simulink model "distributive4"  (R2022b)
settings: Solver=ode8  StartTime=0.0  StopTime=0.25  FixedStep=0.0001  RelTol=1e-3
values from neighbouring files (symbols this model uses):
  A = [a11,0;0,a22]    [distributive3.m]    (also in neurobserver4.m = [1 1;1 2])
  alpha = 0.9e-6    (= 9e-07)    [distributive3.m]
  amp = 80e-6    (= 8e-05)    [distributive3.m]
  angvel = (2*pi)*30    (= 188.495559215)    [distributive3.m]
  B = [b11,0;0,b22]    [distributive3.m]    (also in neurobserver4.m = 1000)
  beta = 0.008    [distributive3.m]
  C = [1,0]    [distributive3.m]
  C_bar = [1,0]    [distributive3.m]    (also in neurobserver4.m = [1,0;0,1])
  d_p = 1.6e-6    (= 1.6e-06)    [distributive3.m]
  fase = 2*pi/10    (= 0.628318530718)    [distributive3.m]
  G = S\C_bar'    [distributive3.m]    (also in neurobserver4.m)
  gamma = 0.008    [distributive3.m]
  Gamma = [0,-B;0 0]    [distributive3.m]    (also in neurobserver4.m = [ 0 , -B ; 0 , 0 ])
  h = legend('Closed-loop response map $(y_d,y)$')    [distributive3.m]    (also in neurobserver4.m = legend('$(y_r,y)$ for $x=7.5$, $f=1Hz$','$(y_r,y)$ for $x=15)
  h_i = 2e-6    (= 2e-06)    [distributive3.m]
  k1 = 7    [distributive3.m]    (also in neurobserver4.m)
  k2 = 7    [distributive3.m]    (also in neurobserver4.m)
  kappa1 = 4e3    (= 4000)    [distributive3.m]    (also in neurobserver4.m = 120)
  L = 20000    [distributive3.m]
  S = [s11,s12;s21,s22]    [distributive3.m]    (also in neurobserver4.m = [1/theta,B/theta^2;B/theta^2,(2*B^2)/theta^3])
  V = learning.V    [neurobserver4.m]
  W = learning.W    [neurobserver4.m]
  x1 = e(2)    [distributive3.m]
  x2 = e(5)    [distributive3.m]
  y_i = -3e-6    (= -3e-06)    [distributive3.m]
undefined symbols (not defined in the file or in its folder): freq, Gamma_c, Y
(part 3 of 3)

== matlab function distributive4/observer10 ==
  data: z_hat input; y input; h_d input; C_bar parameter; S parameter; Gamma parameter; hZ input; z_hat_dot output; V parameter; W parameter
function z_hat_dot   = fcn(z_hat,y,h_d,C_bar,S,Gamma,hZ,V,W)
Y_hat=C_bar'*z_hat;
z=[y;h_d];
Y=C_bar'*z;

sigma = sig_fn(V*hZ);                                              % (8x1) = (8x8)*(8x1)
g_hat = W*sigma;                                                       % hg = (2x1) = (2x8)*(8x1)
G= S\C_bar;
z_hat_dot=Gamma*z_hat + g_hat + G*(Y-Y_hat); %G*C_bar*(z-z_hat); %
end

function [sigvec] = sig_fn(x_vec)
    sigvec = zeros(length(x_vec), 1);
    for i = 1:length(x_vec)
        sigvec(i, 1) = 2/(1 + exp(-2*x_vec(i, 1))) - 1;
    end
end

== matlab function distributive4/observer9 ==
  data: z_hat input; y input; h_d input; C_bar parameter; S parameter; Gamma parameter; hZ input; z_hat_dot output; V parameter; W parameter
function z_hat_dot   = fcn(z_hat,y,h_d,C_bar,S,Gamma,hZ,V,W)
z=[y;h_d];
z_tilde=z-z_hat;

sigma = sig_fn(V*hZ);                                              % (8x1) = (8x8)*(8x1)
g_hat = W*sigma;                                                       % hg = (2x1) = (2x8)*(8x1)
G= S\C_bar;
z_hat_dot=Gamma*z_hat + g_hat + G*(C_bar'*z_tilde); %G*C_bar*(z-z_hat); %
end

function [sigvec] = sig_fn(x_vec)
    sigvec = zeros(length(x_vec), 1);
    for i = 1:length(x_vec)
        sigvec(i, 1) = 2/(1 + exp(-2*x_vec(i, 1))) - 1;
    end
end

== matlab function distributive4/u_ref_dot10 ==
  data: h_d_ref input; z_hat input; u_ref_dot output size=1; alpha parameter size=1; k1 parameter size=1; k2 parameter size=1; x input; L parameter
function u_ref_dot = fcn(h_d_ref,z_hat,alpha,k1,k2,x,L)
h_d_hat=z_hat(2);
% syms c1 c2 k1 k2 alfa betta rho sigma

e = h_d_hat - h_d_ref;
alpha_d=alpha*(x/L)^2;

u_ref_dot=(1/alpha_d)*(k1*sign(e)*sqrt(abs(e)) + k2*e);
%u_ref_dot= k1*sign(e) + k2*e; %este es el ùnico que sí controla el modelo de micky con A_h=0.9e-6

== matlab function distributive4/u_ref_dot11 ==
  data: h_d_ref input; z_hat input; u_ref_dot output size=1; alpha parameter size=1; k1 parameter size=1; k2 parameter size=1; x input; L parameter
function u_ref_dot = fcn(h_d_ref,z_hat,alpha,k1,k2,x,L)
h_d_hat=z_hat(2);
% syms c1 c2 k1 k2 alfa betta rho sigma

e = h_d_hat - h_d_ref;
alpha_d=alpha*(x/L)^2;

u_ref_dot=(1/alpha_d)*(k1*sign(e)*sqrt(abs(e)) + k2*e);
%u_ref_dot= k1*sign(e) + k2*e; %este es el ùnico que sí controla el modelo de micky con A_h=0.9e-6

== matlab function distributive4/v10 ==
  data: d_d input; v output; u input; h_d input
function v = fcn(d_d,u,h_d)

v=d_d*u-h_d;

== matlab function distributive4/Subsystem10/y3 ==
  data: y output; v input; Y input; Y_dot output; A parameter; B parameter; C parameter; t input
function [y,Y_dot] = fcn(v,Y, A, B, C,t)

delta_y = [(30)*t;0];
Y_dot = A*Y + B*v + delta_y;
y=C*Y;

== matlab function distributive4/v11 ==
  data: d_d input; v output; u input; h_d input
function v = fcn(d_d,u,h_d)

v=d_d*u-h_d;

== matlab function distributive4/y12 ==
  data: y output; v input; Y input; Y_dot output; A parameter; B parameter; C parameter
function [y,Y_dot] = fcn(v,Y, A, B, C)
Y_dot=A*Y+B*v;
y=C*Y;

== matlab function distributive4/y13 ==
  data: y output; v input; Y input; Y_dot output; A parameter; B parameter; C parameter
function [y,Y_dot] = fcn(v,Y, A, B, C)
Y_dot=A*Y+B*v;
y=C*Y;

== matlab function distributive4/disturbances ==
  data: t input; delta output
function delta = dist(t)

delta_x = 30e-6; %0;
%delta_h = (25e-6)*sin(t); %0; %2*sin(t);

delta = delta_x;

== matlab function distributive4/dist_vars25/disturbances ==
  data: t input; delta output
function delta = dist(t)


delta_h = (25e-6)*sin(t); %2*sin(t);

delta = delta_h;

== matlab function distributive4/disturbances1 ==
  data: t input; delta output
function delta = dist(t)

delta_x = 30e-6; %0;
%delta_h = (25e-6)*sin(t); %0; %2*sin(t);

delta = delta_x;

== matlab function distributive4/dist_vars24/disturbances ==
  data: t input; delta output
function delta = dist(t)


delta_h = (25e-6)*sin(t); %2*sin(t);

delta = delta_h;

== matlab function distributive4/Subsystem2/Subsystem4/estimator ==
  data: h input; y_d_hat output; h_dot output; h_d_hat output; L parameter; u input; u_dot input; d_p parameter; d_d_hat output; alpha parameter; gamma parameter; x input; beta parameter
function [y_d_hat,h_dot,h_d_hat,d_d_hat]  = fcn(h,L, u,u_dot,d_p, alpha, gamma,x, beta)

d_d_hat = d_p*(x/L)^2;
h_dot = alpha*u_dot - beta*abs(u_dot)*h - gamma*u_dot*abs(h);
%h_d_dot = h_dot*(x/L)^2;
%h_d_hat = h*(x/L)^2;
%u_hat = (y_L + h_d_hat)/d_d_hat;
h_d_hat = h*(x/L)^2;
y_d_hat = d_d_hat*u -h_d_hat;




%h_d=h*(x/L)^2;
%

== matlab function distributive4/Subsystem2/Subsystem4/measurements/MATLAB Function1 ==
  data: h input; u input; y_L output; d_p parameter
function y_L = fcn(h,u,d_p)


y_L = d_p*u-h;

== matlab function distributive4/Subsystem2/Subsystem4/measurements/MATLAB Function5 ==
  data: u_dot input; h_dot output; h input; alpha parameter; gamma parameter; beta parameter
function h_dot = fcn(u_dot,h,alpha, gamma, beta)

h_dot = alpha*u_dot - beta*abs(u_dot)*h - gamma*u_dot*abs(h);

== matlab function distributive4/Subsystem/dist_vars32/MATLAB Function ==
  data: x input; L parameter; d_p parameter; d_d output
function d_d   = fcn(x,L, d_p)

d_d = (x/L)*(x/L)*d_p;

== matlab function distributive4/Subsystem/dist_vars32/MATLAB Function5 ==
  data: u_dot input; h_dot output; h input; x input; alpha parameter; gamma parameter; beta parameter; L parameter; h_d output; t input
function [h_dot,h_d] = fcn(u_dot,h,x,alpha, gamma, beta,L,t)

delta_h=25*t;
h_dot = alpha*u_dot - beta*abs(u_dot)*h - gamma*u_dot*abs(h) + delta_h; % ****
h_d=h*(x/L)^2;     % ****
%h_d_dot = h_dot*(x/L)^2;

% function [h_dot,h_d_dot]  = fcn(u_dot,h,x,alpha, gamma, beta,L,t)

% delta_h=25*t;
% h_dot = alpha*u_dot - beta*abs(u_dot)*h - gamma*u_dot*abs(h) + delta_h;
% h_d_dot = h_dot*(x/L)^2;
%h_d=h*(x/L)^2;

== matlab function distributive4/Subsystem2/inv D3 ==
  data: y_ref input; Y_dot input; A parameter; B parameter; v_ref output; Y output; C parameter
%function h_d_ref = fcn(y,y_ref_dot,d_d,u, A, B)

%y_tilde=y_hat-y_ref;
%h_d_ref=(1/B)*(A*y -y_ref_dot +B*d_d*u);

function [v_ref,Y]  = fcn(y_ref,Y_dot, A, B, C)

Y=y_ref/C;
v_ref = (Y_dot-A*Y)/B;

== matlab function distributive4/dist_vars3/MATLAB Function ==
  data: x input; L parameter; d_p parameter; d_d output
function d_d   = fcn(x,L, d_p)

d_d = (x/L)*(x/L)*d_p;

== matlab function distributive4/Subsystem2/inv v3 ==
  data: v input; h_d input; u_ref output size=1; d_d input size=1
%function u_ref_dot = fcn(h_d_hat,h_d_ref,alpha,k1,k2)
function u_ref = fcn(v,h_d,d_d)
% syms c1 c2 k1 k2 alfa betta rho sigma

%e=h_d_hat-h_d_ref;

%u_ref_dot=(1/alpha)*(-k1*sign(e)*sqrt(abs(e)) -k2*e);

u_ref=(v+h_d)/d_d;

== matlab function distributive4/Subsystem/system v4 ==
  data: d_d input; v output; u input; h_d input; h input; d_p parameter
function v = fcn(d_d,u,h_d,h, d_p)

%v=d_d*u-h_d;
v=[ d_p*u-h ; d_d*u-h_d ];

== matlab function distributive4/Subsystem/y17 ==
  data: y output; v input; Y input; Y_dot output; A parameter; B parameter; C parameter; t input
function [y,Y_dot] = fcn(v,Y, A, B, C,t)
delta_y = (30)*t;
Y_dot = A*Y + B*v + delta_y;
y = C*Y;

% function [y,Y_dot] = fcn(v,Y, A, B, C,t)

% delta_y = (30e-6)*sin(t);
% Y_dot = A*Y + B*v + delta_y;
% y=C*Y;
%

== matlab function distributive4/observer/dist_vars35/MATLAB Function ==
  data: x input; L parameter; d_p parameter; d_d output
function d_d   = fcn(x,L, d_p)

d_d = (x/L)*(x/L)*d_p;

== matlab function distributive4/observer/dist_vars35/MATLAB Function5 ==
  data: u_dot input; h_dot output; h input; x input; alpha parameter; gamma parameter; beta parameter; L parameter; h_d output; h_d_dot output
function [h_dot,h_d,h_d_dot] = fcn(u_dot,h,x,alpha, gamma, beta,L)


h_dot = alpha*u_dot - beta*abs(u_dot)*h - gamma*u_dot*abs(h);
h_d=h*(x/L)^2;
h_d_dot=h_dot*(x/L)^2;

== matlab function distributive4/dist_vars36/MATLAB Function ==
  data: x input; L parameter; d_p parameter; d_d output
function d_d   = fcn(x,L, d_p)

d_d = (x/L)*(x/L)*d_p;

== matlab function distributive4/dist_vars36/MATLAB Function5 ==
  data: u_dot input; h_dot output; h input; x input; alpha parameter; gamma parameter; beta parameter; L parameter; h_d output; h_d_dot output
function [h_dot,h_d,h_d_dot] = fcn(u_dot,h,x,alpha, gamma, beta,L)


h_dot = alpha*u_dot - beta*abs(u_dot)*h - gamma*u_dot*abs(h);
h_d=h*(x/L)^2;
h_d_dot=h_dot*(x/L)^2;

== matlab function distributive4/dist_vars37/MATLAB Function ==
  data: x input; L parameter; d_p parameter; d_d output
function d_d   = fcn(x,L, d_p)

d_d = (x/L)*(x/L)*d_p;

== matlab function distributive4/dist_vars3/MATLAB Function5 ==
  data: u_dot input; h_dot output; h input; x input; alpha parameter; gamma parameter; beta parameter; L parameter; h_d output; h_d_dot output
function [h_dot,h_d,h_d_dot] = fcn(u_dot,h,x,alpha, gamma, beta,L)


h_dot = alpha*u_dot - beta*abs(u_dot)*h - gamma*u_dot*abs(h);
h_d=h*(x/L)^2;
h_d_dot = h_dot*(x/L)^2;

== matlab function distributive4/dist_vars37/MATLAB Function5 ==
  data: u_dot input; h_dot output; h input; x input; alpha parameter; gamma parameter; beta parameter; L parameter; h_d output; h_d_dot output
function [h_dot,h_d,h_d_dot] = fcn(u_dot,h,x,alpha, gamma, beta,L)


h_dot = alpha*u_dot - beta*abs(u_dot)*h - gamma*u_dot*abs(h);
h_d=h*(x/L)^2;
h_d_dot = h_dot*(x/L)^2;

== matlab function distributive4/errors15 ==
  data: z_hat input; y input; h_d input; e_y output; e_h output; e_yr output; e_hr output; y_ref input; h_d_ref input
function [e_y,e_h,e_yr,e_hr]   = fcn(z_hat,y,h_d,y_ref, h_d_ref)
y_d_hat = z_hat(1);
h_d_hat = z_hat(2);
y_d = y(2);


e_y = y_d_hat - y_d;
e_h = h_d_hat - h_d;
e_yr = y_ref - y_d;
e_hr = h_d_ref - h_d;

== matlab function distributive4/errors6 ==
  data: z_hat input; y input; h_d input; e_y output; e_h output; e_yr output; e_hr output; y_ref input; h_d_ref input
function [e_y,e_h,e_yr,e_hr]   = fcn(z_hat,y,h_d,y_ref, h_d_ref)
y_d_hat=z_hat(1);
h_d_hat=z_hat(2);
y_d=y(2);


e_y=y_d_hat-y_d;
e_h=h_d_hat-h_d;
e_yr=y_ref-y_d;
e_hr=h_d_ref-h_d;

== matlab function distributive4/Subsystem6/h_d_ref14 ==
  data: u input; y_ref input; y_ref_dot input; z_hat input; h_d_ref output; A parameter; B parameter; kappa1 parameter; d_d input
function h_d_ref = fcn(u,y_ref, y_ref_dot,z_hat, A, B, kappa1, d_d)

y_hat=z_hat(1); % y_L

y_tilde=y_hat-y_ref;
h_d_ref=B\((A + kappa1)*y_tilde + A*y_ref -y_ref_dot +B*d_d*u);

== matlab function distributive4/h_d_ref15 ==
  data: u input; y_ref input; y_ref_dot input; z_hat input; h_d_ref output; A parameter; B parameter; kappa1 parameter; d_d input
function h_d_ref = fcn(u,y_ref, y_ref_dot,z_hat, A, B, kappa1, d_d)

y_hat=z_hat(1);

y_tilde=y_hat-y_ref;
h_d_ref=B\((A + kappa1)*y_tilde + A*y_ref -y_ref_dot +B*d_d*u);

== matlab function distributive4/observer/observer13 ==
  data: z_hat input; y input; x input; h_d input; C_bar parameter; S parameter; Gamma parameter; hZ input; z_hat_dot output; V parameter; W parameter; L parameter; G parameter
function z_hat_dot   = fcn(z_hat,y,x,h_d,C_bar,S,Gamma,hZ,V,W, L,G)
%y_hat=z_hat(1);
y_L=y(1); % Y=y_L
y_d=y_L*(x/L)^2;
z=[y_d;h_d];


sigma = sigm_fn(V*hZ);                                              % (8x1) = (8x8)*(8x1)
g_hat = W*sigma;                                                       % hg = (2x1) = (2x8)*(8x1)
%G= S\C_bar;

z_hat_dot=Gamma*z_hat + g_hat + G*C_bar*(z-z_hat); %G*C_bar*(z-z_hat); %
end

function [sigvec] = sigm_fn(x_vec)
    sigvec = zeros(length(x_vec), 1);
    for i = 1:length(x_vec)
        sigvec(i, 1) = 2/(1 + exp(-2*x_vec(i, 1))) - 1;
    end
end

== matlab function distributive4/observer14 ==
  data: z_hat input; y input; x input; h_d input; C_bar parameter; S parameter; Gamma parameter; hZ input; z_hat_dot output; V parameter; W parameter; L parameter
function z_hat_dot   = fcn(z_hat,y,x,h_d,C_bar,S,Gamma,hZ,V,W, L)
%y_hat=z_hat(1);
y_L=y(1); % Y=y_L
y_d=y_L*(x/L)^2;
z=[y_d;h_d];


sigma = sigm_fn(V*hZ);                                              % (8x1) = (8x8)*(8x1)
g_hat = W*sigma;                                                       % hg = (2x1) = (2x8)*(8x1)
%G= S\C_bar;

z_hat_dot=Gamma*z_hat + g_hat + S\C_bar*C_bar'*(z-z_hat); %G*C_bar*(z-z_hat); %
end

function [sigvec] = sigm_fn(x_vec)
    sigvec = zeros(length(x_vec), 1);
    for i = 1:length(x_vec)
        sigvec(i, 1) = 2/(1 + exp(-2*x_vec(i, 1))) - 1;
    end
end

== matlab function distributive4/Subsystem6/u_ref_dot14 ==
  data: h_d_ref input; z_hat input; u_ref_dot output size=1; alpha parameter size=1; k1 parameter size=1; k2 parameter size=1; x input; L parameter
function u_ref_dot = fcn(h_d_ref,z_hat,alpha,k1,k2,x,L)
h_d_hat=z_hat(2);
% syms c1 c2 k1 k2 alfa betta rho sigma

e = h_d_hat - h_d_ref;
alpha_d=alpha*(x/L)^2;

u_ref_dot=(1/alpha_d)*(k1*sign(e)*sqrt(abs(e)) + k2*e);
%u_ref_dot= k1*sign(e) + k2*e; %este es el ùnico que sí controla el modelo de micky con A_h=0.9e-6

== matlab function distributive4/u_ref_dot15 ==
  data: h_d_ref input; z_hat input; u_ref_dot output size=1; alpha parameter size=1; k1 parameter size=1; k2 parameter size=1; x input; L parameter
function u_ref_dot = fcn(h_d_ref,z_hat,alpha,k1,k2,x,L)
h_d_hat=z_hat(2);
% syms c1 c2 k1 k2 alfa betta rho sigma

e = h_d_hat - h_d_ref;
alpha_d=alpha*(x/L)^2;

u_ref_dot=(1/alpha_d)*(k1*sign(e)*sqrt(abs(e)) + k2*e);
%u_ref_dot= k1*sign(e) + k2*e; %este es el ùnico que sí controla el modelo de micky con A_h=0.9e-6

== matlab function distributive4/v15 ==
  data: d_d input; h input; v output; u input; h_d input; d_p parameter
function v = fcn(d_d,h,u,h_d, d_p)

v=[ d_p*u-h ; d_d*u-h_d ];

== matlab function distributive4/Subsystem11/h_d_ref14 ==
  data: u input; y_ref input; y_ref_dot input; z_hat input; h_d_ref output; A parameter; B parameter; kappa1 parameter; d_d input
function h_d_ref = fcn(u,y_ref, y_ref_dot,z_hat, A, B, kappa1, d_d)

y_hat=z_hat(1); % y_L

y_tilde=y_hat-y_ref;
h_d_ref=B\((A + kappa1)*y_tilde + A*y_ref -y_ref_dot +B*d_d*u);

== matlab function distributive4/y22 ==
  data: y output; v input; Y input; Y_dot output; A parameter; B parameter; C parameter
function [y,Y_dot] = fcn(v,Y, A, B, C)
Y_dot=A*Y+B*v;
y=C*Y;

== matlab function distributive4/dist_vars39/MATLAB Function ==
  data: x input; L parameter; d_p parameter; d_d output
function d_d   = fcn(x,L, d_p)

d_d = (x/L)*(x/L)*d_p;

== matlab function distributive4/dist_vars39/MATLAB Function5 ==
  data: h_dot output; u_dot input; h input; x input; alpha parameter; gamma parameter; beta parameter; L parameter; h_d_dot output; t input
function [h_dot,h_d_dot]  = fcn(u_dot,h,x,alpha, gamma, beta,L,t)

delta_h=25*t;
h_dot = alpha*u_dot - beta*abs(u_dot)*h - gamma*u_dot*abs(h)+delta_h;
h_d_dot = h_dot*(x/L)^2;
%h_d=h*(x/L)^2;

== matlab function distributive4/dist_vars40/MATLAB Function ==
  data: x input; L parameter; d_p parameter; d_d output
function d_d   = fcn(x,L, d_p)

d_d = (x/L)*(x/L)*d_p;

== matlab function distributive4/dist_vars40/MATLAB Function1 ==
  data: h_dot output; u_dot input; h input; x input; alpha parameter; gamma parameter; beta parameter; L parameter; h_d_dot output
function [h_dot,h_d_dot]  = fcn(u_dot,h,x,alpha, gamma, beta,L)


h_dot = alpha*u_dot - beta*abs(u_dot)*h - gamma*u_dot*abs(h);
h_d_dot = h_dot*(x/L)^2;
%h_d=h*(x/L)^2;

== matlab function distributive4/errors16 ==
  data: z_hat input; y input; h_d input; e_y output; e_h output; e_y2 output; e_h2 output; y_ref input; h_d_ref input
function [e_y,e_h,e_y2,e_h2]   = fcn(z_hat,y,h_d,y_ref, h_d_ref)
e_y=z_hat(1)-y;
e_h=z_hat(2)-h_d;
e_y2=y_ref-y;
e_h2=h_d_ref-h_d;

== matlab function distributive4/observer15 ==
  data: z_hat input; y input; u input; A parameter; B parameter; z_hat_dot output; C_bar parameter; S parameter; Gamma parameter; h_d_dot input size=1; d_d input
function z_hat_dot   = fcn(z_hat,y,u,A, B, C_bar,S,Gamma,h_d_dot,d_d)
y_hat=z_hat(1);
f_hat=h_d_dot;
g_hat=[A*y_hat+B*d_d*u;
        f_hat];
z_hat_dot=Gamma*z_hat + g_hat - (S\C_bar')*(y_hat-y);

== matlab function distributive4/v16 ==
  data: d_d input; v output; u input; h_d input
function v = fcn(d_d,u,h_d)

v=d_d*u-h_d;

== matlab function distributive4/y23 ==
  data: y output; v input; Y input; Y_dot output; A parameter; B parameter; C parameter; t input
function [y,Y_dot] = fcn(v,Y, A, B, C,t)

delta_y=(30e-6)*sin(t);
Y_dot=A*Y+B*v+delta_y;
y=C*Y;

== matlab function distributive4/Subsystem11/u_ref_dot14 ==
  data: h_d_ref input; z_hat input; u_ref_dot output size=1; alpha parameter size=1; k1 parameter size=1; k2 parameter size=1; x input; L parameter
function u_ref_dot = fcn(h_d_ref,z_hat,alpha,k1,k2,x,L)
h_d_hat=z_hat(2);
% syms c1 c2 k1 k2 alfa betta rho sigma

e = h_d_hat - h_d_ref;
alpha_d=alpha*(x/L)^2;

u_ref_dot=(1/alpha_d)*(k1*sign(e)*sqrt(abs(e)) + k2*e);
%u_ref_dot= k1*sign(e) + k2*e; %este es el ùnico que sí controla el modelo de micky con A_h=0.9e-6

== matlab function distributive4/Subsystem12/dist_vars15/MATLAB Function ==
  data: x input; L parameter; d_p parameter; d_d output
function d_d   = fcn(x,L, d_p)

d_d = (x/L)*(x/L)*d_p;

== matlab function distributive4/Subsystem12/dist_vars15/MATLAB Function1 ==
  data: h_dot output; u_dot input; h input; x input; alpha parameter; gamma parameter; beta parameter; L parameter; h_d_dot output
function [h_dot,h_d_dot]  = fcn(u_dot,h,x,alpha, gamma, beta,L)


h_dot = alpha*u_dot - beta*abs(u_dot)*h - gamma*u_dot*abs(h);
h_d_dot = h_dot*(x/L)^2;
%h_d=h*(x/L)^2;

== matlab function distributive4/Subsystem12/observer5 ==
  data: z_hat input; y input; x input; h_d input; u input; A parameter; B parameter; z_hat_dot output; C_bar parameter; S parameter; Gamma parameter; h_d_dot input size=1; d_d input; L parameter; G parameter
function z_hat_dot   = fcn(z_hat,y,x,h_d,u,A, B, C_bar,S,Gamma,h_d_dot,d_d,L,G)
y_L=y(1); % Y=y_L
y_d=y_L*(x/L)^2;
y_hat = z_hat(1);

z=[y_d;h_d];
f_hat = h_d_dot;
g_hat = [A*y_hat + B*d_d*u;
            f_hat         ];
% z_hat_dot = Gamma*z_hat + g_hat - (S\C_bar')*(y_hat-y);  y = Cz



% function z_hat_dot   = fcn(z_hat,y,x,h_d,C_bar,S,Gamma,hZ,V,W, L)
% %y_hat=z_hat(1);
%  y_L=y(1); % Y=y_L
%  y_d=y_L*(x/L)^2;
% z=[y_d;h_d];
                                                   % hg = (2x1) = (2x8)*(8x1)
% G= S\C_bar;
% 
% z_hat_dot = Gamma*z_hat + g_hat + G*C_bar'*(z-z_hat); %G*C_bar*(z-z_hat); %
z_hat_dot = Gamma*z_hat + g_hat + G*C_bar*(z-z_hat); %
% end


% z_hat_dot = Gamma*z_hat + g_hat - (S\C_bar')*(y_hat-y);

== matlab function distributive4/Subsystem8/dist_vars14/MATLAB Function ==
  data: x input; L parameter; d_p parameter; d_d output
function d_d   = fcn(x,L, d_p)

d_d = (x/L)*(x/L)*d_p;

== matlab function distributive4/Subsystem8/dist_vars14/MATLAB Function5 ==
  data: h_dot output; h_d output; u_dot input; h input; x input; alpha parameter; gamma parameter; beta parameter; L parameter; t input
function [h_dot,h_d]  = fcn(u_dot,h,x,alpha, gamma, beta,L,t)

delta_h=25*t;
h_dot = alpha*u_dot - beta*abs(u_dot)*h - gamma*u_dot*abs(h)+delta_h;
%h_d_dot = h_dot*(x/L)^2;
h_d=h*(x/L)^2;

== matlab function distributive4/dist_vars4/MATLAB Function ==
  data: x input; L parameter; d_p parameter; d_d output
function d_d   = fcn(x,L, d_p)

d_d = (x/L)*(x/L)*d_p;

== matlab function distributive4/Subsystem8/v6 ==
  data: d_d input; v output; u input; h_d input; h input; d_p parameter
% function v = fcn(d_d,u,h_d)
% 
% v=d_d*u-h_d;

function v = fcn(d_d,u,h_d,h, d_p)

%v=d_d*u-h_d;
v=[ d_p*u-h ; d_d*u-h_d ];

== matlab function distributive4/Subsystem8/y8 ==
  data: y output; v input; Y input; Y_dot output; A parameter; B parameter; C parameter; t input
function [y,Y_dot] = fcn(v,Y, A, B, C,t)

delta_y = [30*t;0];
Y_dot = A*Y + B*v + delta_y;
y=C*Y;

== matlab function distributive4/Subsystem9/h_d_ref6 ==
  data: u input; Y_ref input; Y_ref_dot input; Y input; h_d_ref output; A parameter; B parameter; kappa1 parameter; d_d input; z_hat input
function h_d_ref = fcn(u,Y_ref, Y_ref_dot,Y, A, B, kappa1, d_d,z_hat)

y_d_hat=z_hat(1);
% Y_tilde=Y(2)-Y_ref; % Y(2)=Y(x)
% Y_tilde=Y(1)-Y_ref; % Y(2)=Y(L)
Y_tilde=y_d_hat-Y_ref; % Y(2)=Y(L)

h_d_ref=B\((A + kappa1)*Y_tilde + A*Y_ref -Y_ref_dot +B*d_d*u);

== matlab function distributive4/Subsystem9/u_ref_dot6 ==
  data: h_d_ref input; z_hat input; u_ref_dot output size=1; alpha parameter size=1; k1 parameter size=1; k2 parameter size=1; x input; L parameter; h_d_dot input
function u_ref_dot = fcn(h_d_ref,z_hat,alpha,k1,k2,x,L,h_d_dot)
h_d_hat=z_hat(2);
% syms c1 c2 k1 k2 alfa betta rho sigma

e_h = h_d_hat - h_d_ref;
alpha_d = alpha*(x/L)^2;

%u_dot =  k1*sign(e) + k2*e; %con este "x" converge mejor ; ver porque debe tener signos [+]
%u_ref_dot= k1*sign(e) + k2*e; %este es el ùnico que sí controla el modelo de micky con A_h=0.9e-6

%u_dot =  (1/A_h)*(-k1*sign(e)*sqrt(abs(e)) - k2*e ); %este tambien

%u_ref_dot=(1/alpha_d)*(-k1*sign(e)*sqrt(abs(e)) - k2*e);
u_ref_dot=(1/alpha_d)*( k1*sign(e_h)*sqrt(abs(e_h)) + k2*e_h );

%u_dot =  (1/A_h)*(- k1*sign(e) - k2*e + hd_dot); % este es el bueno
%u_ref_dot=(1/alpha_d)*(-k1*sign(e) - k2*e + h_d_dot);

== matlab function distributive4/errors1 ==
  data: z_hat input; y input; h_d input; e_y output; e_h output; e_yr output; e_hr output; y_ref input; h_d_ref input
function [e_y,e_h,e_yr,e_hr]   = fcn(z_hat,y,h_d,y_ref, h_d_ref)
y_d_hat=z_hat(1);
h_d_hat=z_hat(2);
y_d=y(2);


e_y=y_d_hat-y_d;
e_h=h_d_hat-h_d;
e_yr=y_ref-y_d;
e_hr=h_d_ref-h_d;

== matlab function distributive4/errors2 ==
  data: z_hat input; y input; h_d input; e_y output; e_h output; e_y2 output; e_h2 output; y_ref input; h_d_ref input
function [e_y,e_h,e_y2,e_h2]   = fcn(z_hat,y,h_d,y_ref, h_d_ref)
e_y=z_hat(1)-y;
e_h=z_hat(2)-h_d;
e_y2=y_ref-y;
e_h2=h_d_ref-h_d;

== matlab function distributive4/h_d_ref1 ==
  data: u input; Y_ref input; Y_ref_dot input; Y input; h_d_ref output; A parameter; B parameter; kappa1 parameter; d_d input
function h_d_ref = fcn(u,Y_ref, Y_ref_dot,Y, A, B, kappa1, d_d)


Y_tilde=Y-Y_ref;
h_d_ref=(1/B)*((A + kappa1)*Y_tilde + A*Y_ref -Y_ref_dot +B*d_d*u);

== matlab function distributive4/observer1 ==
  data: z_hat input; y input; C_bar parameter; S parameter; Gamma_c parameter; hZ input; z_hat_dot output; V parameter; W parameter
function z_hat_dot   = fcn(z_hat,y,C_bar,S,Gamma_c,hZ,V,W)
y_hat=z_hat(1);

%f_hat=h_d_dot;
%g_hat=[A*y_hat+B*d_d*u; f_hat];

%z_tild = z(:, i) - hz(:, i);                                        % state vector: z_tilde = z-z_hat
%y_tild = y - C_bar*z_hat;                                              % output vector: y_tilde = C'x(t)-C'x_hat(t)
%hZ = [v(:, i);z(:, i);dv(:, i);dz(:, i)];                           % (8x1)
%hZ = [v(:, i);dv(2, i)];
%hZ = [v(:, i);z(2, i);dz(2, i)];
sigma = sig_fn(V*hZ);                                              % (8x1) = (8x8)*(8x1)
g_hat = W*sigma;                                                       % hg = (2x1) = (2x8)*(8x1)
%z_hat_dot = Gamma_c*z_hat + hg + G*y_tild;                       % (2x1) = (2x2)*(2x1) + (2x1) + (2x2)*(2x1)   ---> eq 4
%hz(:, i+1) = hz(:, i) + dt*hdz(:, i);                               % x_hat(t+1) = hat_x(t) + dt*x_hat_dot(t)

z_hat_dot=Gamma_c*z_hat + g_hat -S\C_bar'*(y_hat-y);
end

function [sigvec] = sig_fn(x_vec)
    sigvec = zeros(length(x_vec), 1);
    for i = 1:length(x_vec)
        sigvec(i, 1) = 2/(1 + exp(-2*x_vec(i, 1))) - 1;
    end
end

== matlab function distributive4/errors3 ==
  data: z_hat input; y input; h_d input; e_y output; e_h output; e_y2 output; e_h2 output; y_ref input; h_d_ref input
function [e_y,e_h,e_y2,e_h2]   = fcn(z_hat,y,h_d,y_ref, h_d_ref)
e_y=z_hat(1)-y;
e_h=z_hat(2)-h_d;
e_y2=y_ref-y;
e_h2=h_d_ref-h_d;

== matlab function distributive4/estimator1 ==
  data: x input; h input; y_d_hat output; u_hat output; h_d_hat output; L parameter; u input; d_p parameter; d_d_hat output; y_L input
function [y_d_hat,u_hat,h_d_hat,d_d_hat]  = fcn(x,h,L, u,d_p,y_L)

d_d_hat = d_p*(x/L)^2;
h_d_hat = h*(x/L)^2;
u_hat = (y_L + h_d_hat)/d_d_hat;
y_d_hat = d_d_hat*u -h_d_hat;

== matlab function distributive4/measurements1/MATLAB Function1 ==
  data: h input; u input; y_L output; d_p parameter
function y_L = fcn(h,u,d_p)




y_L = d_p*u-h;

== matlab function distributive4/h_d_ref2 ==
  data: u input; Y_ref input; Y_ref_dot input; Y input; h_d_ref output; A parameter; B parameter; d_d input; kappa1 parameter
function h_d_ref = fcn(u,Y_ref, Y_ref_dot,Y, A, B, d_d,kappa1)



Y_tilde=Y-Y_ref;
h_d_ref=B\((A + kappa1)*Y_tilde + A*Y_ref -Y_ref_dot +B*d_d*u);

== matlab function distributive4/measurements1/MATLAB Function5 ==
  data: u_dot input; h_dot output; h input; alpha parameter; gamma parameter; beta parameter
function h_dot = fcn(u_dot,h,alpha, gamma, beta)

h_dot = alpha*u_dot - beta*abs(u_dot)*h - gamma*u_dot*abs(h);

== matlab function distributive4/u_ref_dot2 ==
  data: h_d_ref input; h_d_hat input; u_ref_dot output size=1; alpha parameter size=1; k1 parameter size=1; k2 parameter size=1
function u_ref_dot = fcn(h_d_ref,h_d_hat,alpha,k1,k2)
%h_d_hat=z_hat(2);
% syms c1 c2 k1 k2 alfa betta rho sigma

e=h_d_hat-h_d_ref;

u_ref_dot=(1/alpha)*(-k1*sign(e)*sqrt(abs(e)) -k2*e);

== matlab function distributive4/Subsystem5/dist_vars1/MATLAB Function ==
  data: x input; L parameter; d_p parameter; d_d output
function d_d   = fcn(x,L, d_p)

d_d = (x/L)*(x/L)*d_p;

== matlab function distributive4/v2 ==
  data: d_d input; v output; u input; h_d input
function v = fcn(d_d,u,h_d)

v=d_d*u-h_d;

== matlab function distributive4/y2 ==
  data: y output; v input; Y input; Y_dot output; A parameter; B parameter; C parameter
function [y,Y_dot] = fcn(v,Y, A, B, C)
Y_dot=A*Y+B*v;
y=C*Y;

== matlab function distributive4/observer2/dist_vars35/MATLAB Function ==
  data: x input; L parameter; d_p parameter; d_d output
function d_d   = fcn(x,L, d_p)

d_d = (x/L)*(x/L)*d_p;

== matlab function distributive4/dist_vars6/MATLAB Function ==
  data: x input; L parameter; d_p parameter; d_d output
function d_d   = fcn(x,L, d_p)

d_d = (x/L)*(x/L)*d_p;

== matlab function distributive4/dist_vars6/MATLAB Function5 ==
  data: u_dot input; h_dot output; h input; x input; alpha parameter; gamma parameter; beta parameter; L parameter; h_d output; h_d_dot output
function [h_dot,h_d,h_d_dot] = fcn(u_dot,h,x,alpha, gamma, beta,L)


h_dot = alpha*u_dot - beta*abs(u_dot)*h - gamma*u_dot*abs(h);
h_d=h*(x/L)^2;
h_d_dot = h_dot*(x/L)^2;

== matlab function distributive4/observer2/dist_vars35/MATLAB Function5 ==
  data: u_dot input; h_dot output; h input; x input; alpha parameter; gamma parameter; beta parameter; L parameter; h_d output; h_d_dot output
function [h_dot,h_d,h_d_dot] = fcn(u_dot,h,x,alpha, gamma, beta,L)


h_dot = alpha*u_dot - beta*abs(u_dot)*h - gamma*u_dot*abs(h);
h_d=h*(x/L)^2;
h_d_dot=h_dot*(x/L)^2;

== matlab function distributive4/u_ref_dot1 ==
  data: h_d_ref input; z_hat input; u_ref_dot output size=1; alpha parameter size=1; k1 parameter size=1; k2 parameter size=1
function u_ref_dot = fcn(h_d_ref,z_hat,alpha,k1,k2)
h_d_hat=z_hat(2);
% syms c1 c2 k1 k2 alfa betta rho sigma

e = h_d_hat - h_d_ref;

u_ref_dot=(1/alpha)*(-k1*sign(e)*sqrt(abs(e)) - k2*e);

== matlab function distributive4/v1 ==
  data: d_d input; v output; u input; h_d input
function v = fcn(d_d,u,h_d)

v=d_d*u-h_d;

== matlab function distributive4/Subsystem5/dist_vars1/MATLAB Function5 ==
  data: h_dot output; h_d output; u_dot input; h input; x input; alpha parameter; gamma parameter; beta parameter; L parameter; t input
function [h_dot,h_d]  = fcn(u_dot,h,x,alpha, gamma, beta,L,t)

delta_h=25*t;
h_dot = alpha*u_dot - beta*abs(u_dot)*h - gamma*u_dot*abs(h)+delta_h;
%h_d_dot = h_dot*(x/L)^2;
h_d=h*(x/L)^2;

== matlab function distributive4/y1 ==
  data: y output; v input; Y input; Y_dot output; A parameter; B parameter; C parameter
function [y,Y_dot] = fcn(v,Y, A, B, C)
Y_dot=A*Y+B*v;
y=C*Y;

== matlab function distributive4/observer2/observer13 ==
  data: z_hat input; y input; x input; h_d input; C_bar parameter; S parameter; Gamma parameter; hZ input; z_hat_dot output; V parameter; W parameter; L parameter; G parameter
function z_hat_dot   = fcn(z_hat,y,x,h_d,C_bar,S,Gamma,hZ,V,W, L,G)
%y_hat=z_hat(1);
y_L=y(1); % Y=y_L
y_d=y_L*(x/L)^2;
z=[y_d;h_d];


sigma = sigm_fn(V*hZ);                                              % (8x1) = (8x8)*(8x1)
g_hat = W*sigma;                                                       % hg = (2x1) = (2x8)*(8x1)
%G= S\C_bar;

z_hat_dot=Gamma*z_hat + g_hat + G*C_bar*(z-z_hat); %G*C_bar*(z-z_hat); %
end

function [sigvec] = sigm_fn(x_vec)
    sigvec = zeros(length(x_vec), 1);
    for i = 1:length(x_vec)
        sigvec(i, 1) = 2/(1 + exp(-2*x_vec(i, 1))) - 1;
    end
end

== matlab function distributive4/Subsystem13/dist_vars1/MATLAB Function ==
  data: x input; L parameter; d_p parameter; d_d output
function d_d   = fcn(x,L, d_p)

d_d = (x/L)*(x/L)*d_p;

== matlab function distributive4/Subsystem13/dist_vars1/MATLAB Function5 ==
  data: h_dot output; h_d output; u_dot input; h input; x input; alpha parameter; gamma parameter; beta parameter; L parameter; t input
function [h_dot,h_d]  = fcn(u_dot,h,x,alpha, gamma, beta,L,t)

delta_h=25*t;
h_dot = alpha*u_dot - beta*abs(u_dot)*h - gamma*u_dot*abs(h)+delta_h;
%h_d_dot = h_dot*(x/L)^2;
h_d=h*(x/L)^2;

== matlab function distributive4/Subsystem13/v3 ==
  data: d_d input; v output; u input; h_d input; h input; d_p parameter
% function v = fcn(d_d,u,h_d)
% 
% v=d_d*u-h_d;

function v = fcn(d_d,u,h_d,h, d_p)

%v=d_d*u-h_d;
v=[ d_p*u-h ; d_d*u-h_d ];

== matlab function distributive4/Subsystem13/y3 ==
  data: y output; v input; Y input; Y_dot output; A parameter; B parameter; C parameter; t input
function [y,Y_dot] = fcn(v,Y, A, B, C,t)

delta_y = [(30);0];
Y_dot = A*Y + B*v + delta_y;
y=C*Y;

== matlab function distributive4/Subsystem14/h_d_ref14 ==
  data: u input; y_ref input; y_ref_dot input; z_hat input; h_d_ref output; A parameter; B parameter; kappa1 parameter; d_d input
function h_d_ref = fcn(u,y_ref, y_ref_dot,z_hat, A, B, kappa1, d_d)

y_hat=z_hat(1); % y_L

y_tilde=y_hat-y_ref;
h_d_ref=B\((A + kappa1)*y_tilde + A*y_ref -y_ref_dot +B*d_d*u);

== matlab function distributive4/Subsystem14/u_ref_dot14 ==
  data: h_d_ref input; z_hat input; u_ref_dot output size=1; alpha parameter size=1; k1 parameter size=1; k2 parameter size=1; x input; L parameter
function u_ref_dot = fcn(h_d_ref,z_hat,alpha,k1,k2,x,L)
h_d_hat=z_hat(2);
% syms c1 c2 k1 k2 alfa betta rho sigma

e = h_d_hat - h_d_ref;
alpha_d=alpha*(x/L)^2;

u_ref_dot=(1/alpha_d)*(k1*sign(e)*sqrt(abs(e)) + k2*e);
%u_ref_dot= k1*sign(e) + k2*e; %este es el ùnico que sí controla el modelo de micky con A_h=0.9e-6

== matlab function distributive4/Subsystem1/estimator ==
  data: h input; y_d_hat output; h_dot output; h_d_hat output; L parameter; u input; u_dot input; d_p parameter; d_d_hat output; alpha parameter; gamma parameter; x input; beta parameter
function [y_d_hat,h_dot,h_d_hat,d_d_hat]  = fcn(h,L, u,u_dot,d_p, alpha, gamma,x, beta)

d_d_hat = d_p*(x/L)^2;
h_dot = alpha*u_dot - beta*abs(u_dot)*h - gamma*u_dot*abs(h);
%h_d_dot = h_dot*(x/L)^2;
%h_d_hat = h*(x/L)^2;
%u_hat = (y_L + h_d_hat)/d_d_hat;
h_d_hat = h*(x/L)^2;
y_d_hat = d_d_hat*u -h_d_hat;




%h_d=h*(x/L)^2;
%

== matlab function distributive4/Subsystem15/dist_vars15/MATLAB Function ==
  data: x input; L parameter; d_p parameter; d_d output
function d_d   = fcn(x,L, d_p)

d_d = (x/L)*(x/L)*d_p;

== matlab function distributive4/Subsystem15/dist_vars15/MATLAB Function1 ==
  data: h_dot output; u_dot input; h input; x input; alpha parameter; gamma parameter; beta parameter; L parameter; h_d_dot output
function [h_dot,h_d_dot]  = fcn(u_dot,h,x,alpha, gamma, beta,L)


h_dot = alpha*u_dot - beta*abs(u_dot)*h - gamma*u_dot*abs(h);
h_d_dot = h_dot*(x/L)^2;
%h_d=h*(x/L)^2;

== matlab function distributive4/Subsystem15/observer5 ==
  data: z_hat input; y input; x input; h_d input; u input; A parameter; B parameter; z_hat_dot output; C_bar parameter; S parameter; Gamma parameter; h_d_dot input size=1; d_d input; L parameter; G parameter
function z_hat_dot   = fcn(z_hat,y,x,h_d,u,A, B, C_bar,S,Gamma,h_d_dot,d_d,L,G)
y_L=y(1); % Y=y_L
y_d=y_L*(x/L)^2;
y_hat = z_hat(1);

z=[y_d;h_d];
f_hat = h_d_dot;
g_hat = [A*y_hat + B*d_d*u;
            f_hat         ];
% z_hat_dot = Gamma*z_hat + g_hat - (S\C_bar')*(y_hat-y);  y = Cz



% function z_hat_dot   = fcn(z_hat,y,x,h_d,C_bar,S,Gamma,hZ,V,W, L)
% %y_hat=z_hat(1);
%  y_L=y(1); % Y=y_L
%  y_d=y_L*(x/L)^2;
% z=[y_d;h_d];
                                                   % hg = (2x1) = (2x8)*(8x1)
% G= S\C_bar;
% 
% z_hat_dot = Gamma*z_hat + g_hat + G*C_bar'*(z-z_hat); %G*C_bar*(z-z_hat); %
z_hat_dot = Gamma*z_hat + g_hat + G*C_bar*(z-z_hat); %
% end


% z_hat_dot = Gamma*z_hat + g_hat - (S\C_bar')*(y_hat-y);

== matlab function distributive4/Subsystem5/v3 ==
  data: d_d input; v output; u input; h_d input; h input; d_p parameter
% function v = fcn(d_d,u,h_d)
% 
% v=d_d*u-h_d;

function v = fcn(d_d,u,h_d,h, d_p)

%v=d_d*u-h_d;
v=[ d_p*u-h ; d_d*u-h_d ];

== matlab function distributive4/Subsystem16/dist_vars14/MATLAB Function ==
  data: x input; L parameter; d_p parameter; d_d output
function d_d   = fcn(x,L, d_p)

d_d = (x/L)*(x/L)*d_p;

== matlab function distributive4/Subsystem1/measurements/MATLAB Function1 ==
  data: h input; u input; y_L output; d_p parameter
function y_L = fcn(h,u,d_p)


y_L = d_p*u-h;

== matlab function distributive4/Subsystem1/measurements/MATLAB Function5 ==
  data: u_dot input; h_dot output; h input; alpha parameter; gamma parameter; beta parameter
function h_dot = fcn(u_dot,h,alpha, gamma, beta)

h_dot = alpha*u_dot - beta*abs(u_dot)*h - gamma*u_dot*abs(h);

== matlab function distributive4/dist_vars11/MATLAB Function ==
  data: x input; L parameter; d_p parameter; d_d output
function d_d   = fcn(x,L, d_p)

d_d = (x/L)*(x/L)*d_p;

== matlab function distributive4/dist_vars11/MATLAB Function5 ==
  data: u_dot input; h_dot output; h input; x input; alpha parameter; gamma parameter; beta parameter; L parameter; h_d output; h_d_dot output
function [h_dot,h_d,h_d_dot] = fcn(u_dot,h,x,alpha, gamma, beta,L)


h_dot = alpha*u_dot - beta*abs(u_dot)*h - gamma*u_dot*abs(h);
h_d=h*(x/L)^2;
h_d_dot = h_dot*(x/L)^2;

== matlab function distributive4/errors4 ==
  data: z_hat input; y input; h_d input; e_y output; e_h output; e_y2 output; e_h2 output; y_ref input; h_d_ref input
function [e_y,e_h,e_y2,e_h2]   = fcn(z_hat,y,h_d,y_ref, h_d_ref)
e_y=z_hat(1)-y;
e_h=z_hat(2)-h_d;
e_y2=y_ref-y;
e_h2=h_d_ref-h_d;

== matlab function distributive4/Subsystem16/dist_vars14/MATLAB Function5 ==
  data: h_dot output; h_d output; u_dot input; h input; x input; alpha parameter; gamma parameter; beta parameter; L parameter; t input
function [h_dot,h_d]  = fcn(u_dot,h,x,alpha, gamma, beta,L,t)

delta_h=25*t;
h_dot = alpha*u_dot - beta*abs(u_dot)*h - gamma*u_dot*abs(h)+delta_h;
%h_d_dot = h_dot*(x/L)^2;
h_d=h*(x/L)^2;

== matlab function distributive4/Subsystem16/v6 ==
  data: d_d input; v output; u input; h_d input; h input; d_p parameter
% function v = fcn(d_d,u,h_d)
% 
% v=d_d*u-h_d;

function v = fcn(d_d,u,h_d,h, d_p)

%v=d_d*u-h_d;
v=[ d_p*u-h ; d_d*u-h_d ];

== matlab function distributive4/system v1 ==
  data: d_d input; v output; u input; h_d input
function v = fcn(d_d,u,h_d)

v=d_d*u-h_d;

== matlab function distributive4/Subsystem5/y3 ==
  data: y output; v input; Y input; Y_dot output; A parameter; B parameter; C parameter; t input
function [y,Y_dot] = fcn(v,Y, A, B, C,t)

delta_y = [(30);0];
Y_dot = A*Y + B*v + delta_y;
y=C*Y;

== matlab function distributive4/y5 ==
  data: y output; v input; Y input; Y_dot output; A parameter; B parameter; C parameter
function [y,Y_dot] = fcn(v,Y, A, B, C)
Y_dot=A*Y + B*v;
y=C*Y;

== matlab function distributive4/Subsystem16/y8 ==
  data: y output; v input; Y input; Y_dot output; A parameter; B parameter; C parameter; t input
function [y,Y_dot] = fcn(v,Y, A, B, C,t)

delta_y = [30*t;0];
Y_dot = A*Y + B*v + delta_y;
y=C*Y;

== matlab function distributive4/Subsystem17/h_d_ref6 ==
  data: u input; Y_ref input; Y_ref_dot input; Y input; h_d_ref output; A parameter; B parameter; kappa1 parameter; d_d input; z_hat input
function h_d_ref = fcn(u,Y_ref, Y_ref_dot,Y, A, B, kappa1, d_d,z_hat)

y_d_hat=z_hat(1);
% Y_tilde=Y(2)-Y_ref; % Y(2)=Y(x)
% Y_tilde=Y(1)-Y_ref; % Y(2)=Y(L)
Y_tilde=y_d_hat-Y_ref; % Y(2)=Y(L)

h_d_ref=B\((A + kappa1)*Y_tilde + A*Y_ref -Y_ref_dot +B*d_d*u);

== matlab function distributive4/Subsystem17/u_ref_dot6 ==
  data: h_d_ref input; z_hat input; u_ref_dot output size=1; alpha parameter size=1; k1 parameter size=1; k2 parameter size=1; x input; L parameter; h_d_dot input
function u_ref_dot = fcn(h_d_ref,z_hat,alpha,k1,k2,x,L,h_d_dot)
h_d_hat=z_hat(2);
% syms c1 c2 k1 k2 alfa betta rho sigma

e_h = h_d_hat - h_d_ref;
alpha_d = alpha*(x/L)^2;

%u_dot =  k1*sign(e) + k2*e; %con este "x" converge mejor ; ver porque debe tener signos [+]
%u_ref_dot= k1*sign(e) + k2*e; %este es el ùnico que sí controla el modelo de micky con A_h=0.9e-6

%u_dot =  (1/A_h)*(-k1*sign(e)*sqrt(abs(e)) - k2*e ); %este tambien

%u_ref_dot=(1/alpha_d)*(-k1*sign(e)*sqrt(abs(e)) - k2*e);
u_ref_dot=(1/alpha_d)*( k1*sign(e_h)*sqrt(abs(e_h)) + k2*e_h );

%u_dot =  (1/A_h)*(- k1*sign(e) - k2*e + hd_dot); % este es el bueno
%u_ref_dot=(1/alpha_d)*(-k1*sign(e) - k2*e + h_d_dot);

== matlab function distributive4/errors5 ==
  data: z_hat input; y input; h_d input; e_y output; e_h output; e_yr output; e_hr output; y_ref input; h_d_ref input
function [e_y,e_h,e_yr,e_hr]   = fcn(z_hat,y,h_d,y_ref, h_d_ref)
y_d_hat = z_hat(1);
h_d_hat = z_hat(2);
y_d=y(2); % y(x)


e_y = y_d_hat - y_d;
e_h = h_d_hat - h_d;
e_yr = y_ref - y_d;
e_hr = h_d_ref - h_d;

== matlab function distributive4/errors8 ==
  data: z_hat input; y input; h_d input; e_y output; e_h output; e_y2 output; e_h2 output; y_ref input; h_d_ref input
function [e_y,e_h,e_y2,e_h2]   = fcn(z_hat,y,h_d,y_ref, h_d_ref)
e_y=z_hat(1)-y(2);
e_h=z_hat(2)-h_d;
e_y2=y_ref-y(2);
e_h2=h_d_ref-h_d;

== matlab function distributive4/observer3/dist_vars35/MATLAB Function ==
  data: x input; L parameter; d_p parameter; d_d output
function d_d   = fcn(x,L, d_p)

d_d = (x/L)*(x/L)*d_p;

== matlab function distributive4/observer3/dist_vars35/MATLAB Function5 ==
  data: u_dot input; h_dot output; h input; x input; alpha parameter; gamma parameter; beta parameter; L parameter; h_d output; h_d_dot output
function [h_dot,h_d,h_d_dot] = fcn(u_dot,h,x,alpha, gamma, beta,L)


h_dot = alpha*u_dot - beta*abs(u_dot)*h - gamma*u_dot*abs(h);
h_d=h*(x/L)^2;
h_d_dot=h_dot*(x/L)^2;

== matlab function distributive4/observer3/observer13 ==
  data: z_hat input; y input; x input; h_d input; C_bar parameter; S parameter; Gamma parameter; hZ input; z_hat_dot output; V parameter; W parameter; L parameter; G parameter
function z_hat_dot   = fcn(z_hat,y,x,h_d,C_bar,S,Gamma,hZ,V,W, L,G)
%y_hat=z_hat(1);
y_L=y(1); % Y=y_L
y_d=y_L*(x/L)^2;
z=[y_d;h_d];


sigma = sigm_fn(V*hZ);                                              % (8x1) = (8x8)*(8x1)
g_hat = W*sigma;                                                       % hg = (2x1) = (2x8)*(8x1)
%G= S\C_bar;

z_hat_dot=Gamma*z_hat + g_hat + G*C_bar*(z-z_hat); %G*C_bar*(z-z_hat); %
end

function [sigvec] = sigm_fn(x_vec)
    sigvec = zeros(length(x_vec), 1);
    for i = 1:length(x_vec)
        sigvec(i, 1) = 2/(1 + exp(-2*x_vec(i, 1))) - 1;
    end
end

== matlab function distributive4/Subsystem10/dist_vars1/MATLAB Function ==
  data: x input; L parameter; d_p parameter; d_d output
function d_d   = fcn(x,L, d_p)

d_d = (x/L)*(x/L)*d_p;

== matlab function distributive4/Subsystem3/dist_vars14/MATLAB Function ==
  data: x input; L parameter; d_p parameter; d_d output
function d_d   = fcn(x,L, d_p)

d_d = (x/L)*(x/L)*d_p;

== matlab function distributive4/Subsystem3/dist_vars14/MATLAB Function5 ==
  data: h_dot output; h_d output; u_dot input; h input; x input; alpha parameter; gamma parameter; beta parameter; L parameter; t input
function [h_dot,h_d]  = fcn(u_dot,h,x,alpha, gamma, beta,L,t)

delta_h=25*t;
h_dot = alpha*u_dot - beta*abs(u_dot)*h - gamma*u_dot*abs(h)+delta_h;
%h_d_dot = h_dot*(x/L)^2;
h_d=h*(x/L)^2;

== matlab function distributive4/Subsystem7/dist_vars15/MATLAB Function ==
  data: x input; L parameter; d_p parameter; d_d output
function d_d   = fcn(x,L, d_p)

d_d = (x/L)*(x/L)*d_p;

== matlab function distributive4/Subsystem7/dist_vars15/MATLAB Function1 ==
  data: h_dot output; u_dot input; h input; x input; alpha parameter; gamma parameter; beta parameter; L parameter; h_d_dot output
function [h_dot,h_d_dot]  = fcn(u_dot,h,x,alpha, gamma, beta,L)


h_dot = alpha*u_dot - beta*abs(u_dot)*h - gamma*u_dot*abs(h);
h_d_dot = h_dot*(x/L)^2;
%h_d=h*(x/L)^2;

== matlab function distributive4/errors7 ==
  data: z_hat input; y input; h_d input; e_y output; e_h output; e_y2 output; e_h2 output; y_ref input; h_d_ref input
function [e_y,e_h,e_y2,e_h2]   = fcn(z_hat,y,h_d,y_ref, h_d_ref)
e_y=z_hat(1)-y(2); % y_hat - y_d 
e_h=z_hat(2)-h_d;   % h_hat - h_d
e_y2=y_ref-y(2);
e_h2=h_d_ref-h_d;

== matlab function distributive4/Subsystem4/h_d_ref6 ==
  data: u input; Y_ref input; Y_ref_dot input; Y input; h_d_ref output; A parameter; B parameter; kappa1 parameter; d_d input; z_hat input
function h_d_ref = fcn(u,Y_ref, Y_ref_dot,Y, A, B, kappa1, d_d,z_hat)

y_d_hat=z_hat(1);
% Y_tilde=Y(2)-Y_ref; % Y(2)=Y(x)
% Y_tilde=Y(1)-Y_ref; % Y(2)=Y(L)
Y_tilde=y_d_hat-Y_ref; % Y(2)=Y(L)

h_d_ref=B\((A + kappa1)*Y_tilde + A*Y_ref -Y_ref_dot +B*d_d*u);
